simulink model "simulation_scalar_robustness"  (R2021b)
settings: Solver=VariableStepAuto  StartTime=0.0  StopTime=20  MaxStep=0.01  RelTol=1e-3
values from neighbouring files (symbols this model uses):
  Delta = [1.9 0 -0.5 0 0.3 0 0.8 1.2 0 0 0 0 ... (25 elements, 5x5)]    [robustness.mat]    (also in test_URSR.m = round(Delta,1))
  k43 = 0    [exception.mat]    (also in robustness.mat = 663.324958071; scalar.mat = 61.6408497202; scalar_net.m = sqrt(2)*omega43*sqrt(abs(M(4,3)/M(3,4))); scalar_net_CreationNewConnection.m = sqrt(2)*omega43*sqrt(abs(M(4,3)/M(3,4))))
  k51 = 946.044396421    [exception.mat]    (also in robustness.mat = 146.385010942; scalar.mat = 259.670461528; scalar_net.m = sqrt(2)*omega51*sqrt(abs(M(5,1)/M(1,5))); scalar_net_CreationNewConnection.m = sqrt(2)*omega51*sqrt(abs(M(5,1)/M(1,5))))
  M = [-1.5 0 -0.7 0 17.9 0 -4.1 -6.8 0 0 0 0 ... (25 elements, 5x5)]    [exception.mat]    (also in nonscalar.mat = [-3.8 1.9 -4.5 0 0 0 -4.6 1.6 0 0 0 0 ... (25 elements, 5x5); nonscalar_net.m = round(M,1); nonscalar_net_general.m = sym('M',sum(n)); robustness.mat = [-8.5 0 -1.6 0 1.5 0 -5.3 -4.7 0 0 0 0 ... (25 elements, 5x5)
  omega43 = 50    [exception.mat]    (also in robustness.mat; scalar.mat; scalar_net.m = 200; scalar_net_CreationNewConnection.m)
  omega51 = 50    [exception.mat]    (also in robustness.mat = 70.7106781187; scalar.mat = 70.7106781187; scalar_net.m = sqrt(2) * omega_0; scalar_net_CreationNewConnection.m = sqrt(2) * omega_0)
  T = 2    [robustness.mat]    (also in test_URSR.m = -1/max(real(eig_M))*2*pi)
  x_0 = [1 1 1 1 1]    [exception.mat]    (also in nonscalar_net.m = ones(sum(n),1); robustness.mat; scalar.mat; scalar_net.m = ones(5,1))
settings Model: Creator=alber  LastModifiedBy=anobili

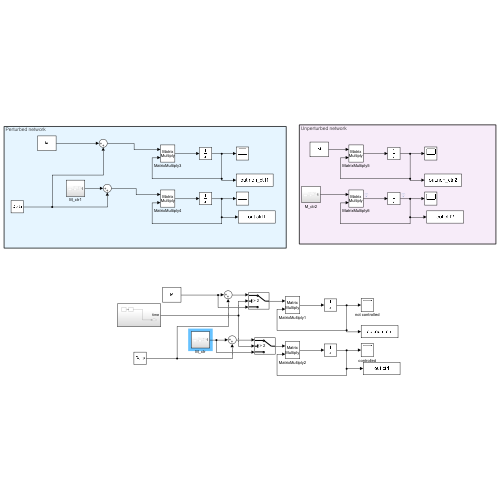
[thumbnail: Simulink's stored preview of the top-level diagram]
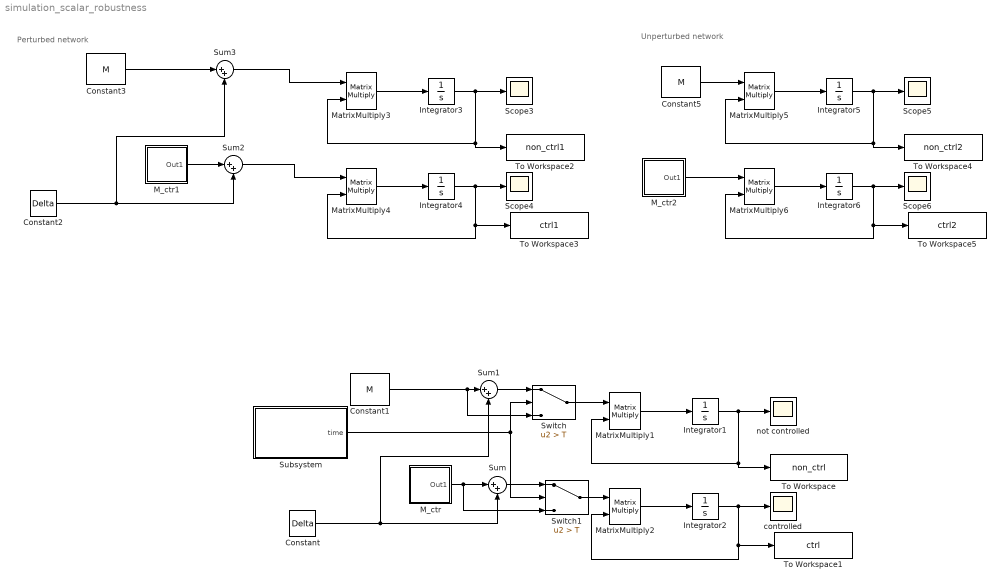
== system simulation_scalar_robustness ==
  note: Perturbed network
  note: Unperturbed network
  Constant : Constant  Value=Delta
  Constant1 : Constant  Value=M
  Constant2 : Constant  Value=Delta
  Constant3 : Constant  Value=M
  Constant5 : Constant  Value=M
  Integrator{1..6} (6 alike) : Integrator  InitialCondition=x_0
  M_ctr : Subsystem
  M_ctr1 : Subsystem
  M_ctr2 : Subsystem
  MatrixMultiply{1..6} (6 alike) : Product  Multiplication=Matrix(*)
  Scope{3..6} (4 alike) : Scope
  Subsystem : Subsystem
  Sum{,1..3} (4 alike) : Sum  Inputs=|++
  Switch : Switch  Criteria=u2 > Threshold  Threshold=T
  Switch1 : Switch  Criteria=u2 > Threshold  Threshold=T
  To Workspace : ToWorkspace  VariableName=non_ctrl  SaveFormat=Timeseries  SampleTime=-1
  To Workspace1 : ToWorkspace  VariableName=ctrl  SaveFormat=Timeseries  SampleTime=-1
  To Workspace2 : ToWorkspace  VariableName=non_ctrl1  SaveFormat=Timeseries  SampleTime=-1
  To Workspace3 : ToWorkspace  VariableName=ctrl1  SaveFormat=Timeseries  SampleTime=-1
  To Workspace4 : ToWorkspace  VariableName=non_ctrl2  SaveFormat=Timeseries  SampleTime=-1
  To Workspace5 : ToWorkspace  VariableName=ctrl2  SaveFormat=Timeseries  SampleTime=-1
  controlled : Scope
  not controlled : Scope
  wires:
  MatrixMultiply1/1 -> Integrator1/1
  Constant1/1 -> Switch/3, Sum1/1
  Integrator1/1 -> not controlled/1, To Workspace/1, MatrixMultiply1/2
  Integrator2/1 -> controlled/1, To Workspace1/1, MatrixMultiply2/2
  MatrixMultiply2/1 -> Integrator2/1
  Switch/1 -> MatrixMultiply1/1
  Switch1/1 -> MatrixMultiply2/1
  M_ctr/1(Out1) -> Switch1/3, Sum/1
  Subsystem/1(time) -> Switch1/2, Switch/2
  Constant/1 -> Sum1/2, Sum/2
  Sum1/1 -> Switch/1
  Sum/1 -> Switch1/1
  Sum2/1 -> MatrixMultiply4/1
  MatrixMultiply4/1 -> Integrator4/1
  Constant3/1 -> Sum3/1
  MatrixMultiply3/1 -> Integrator3/1
  Integrator3/1 -> Scope3/1, To Workspace2/1, MatrixMultiply3/2
  M_ctr1/1(Out1) -> Sum2/1
  Sum3/1 -> MatrixMultiply3/1
  Integrator4/1 -> Scope4/1, To Workspace3/1, MatrixMultiply4/2
  Constant2/1 -> Sum3/2, Sum2/2
  M_ctr2/1(Out1) -> MatrixMultiply6/1
  Integrator6/1 -> Scope6/1, To Workspace5/1, MatrixMultiply6/2
  Constant5/1 -> MatrixMultiply5/1
  Integrator5/1 -> Scope5/1, To Workspace4/1, MatrixMultiply5/2
  MatrixMultiply5/1 -> Integrator5/1
  MatrixMultiply6/1 -> Integrator6/1

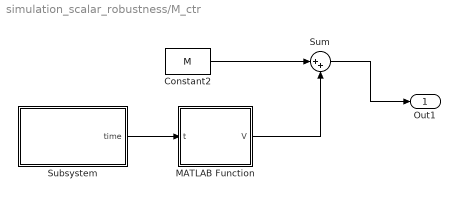
== system simulation_scalar_robustness/M_ctr ==
  Constant2 : Constant  Value=M
  MATLAB Function : MATLAB Function  TreatAsAtomicUnit=on
  Subsystem : Subsystem
  Sum : Sum  Inputs=|++
  Out1 : Outport
  wires:
  Constant2/1 -> Sum/1
  MATLAB Function/1(V) -> Sum/2
  Subsystem/1(time) -> MATLAB Function/1(t)
  Sum/1 -> Out1/1

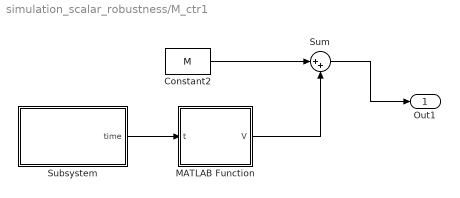
== system simulation_scalar_robustness/M_ctr1 ==
  Constant2 : Constant  Value=M
  MATLAB Function : MATLAB Function  TreatAsAtomicUnit=on
  Subsystem : Subsystem
  Sum : Sum  Inputs=|++
  Out1 : Outport
  wires:
  Constant2/1 -> Sum/1
  MATLAB Function/1(V) -> Sum/2
  Subsystem/1(time) -> MATLAB Function/1(t)
  Sum/1 -> Out1/1

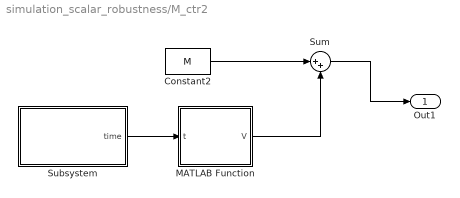
== system simulation_scalar_robustness/M_ctr2 ==
  Constant2 : Constant  Value=M
  MATLAB Function : MATLAB Function  TreatAsAtomicUnit=on
  Subsystem : Subsystem
  Sum : Sum  Inputs=|++
  Out1 : Outport
  wires:
  Constant2/1 -> Sum/1
  MATLAB Function/1(V) -> Sum/2
  Subsystem/1(time) -> MATLAB Function/1(t)
  Sum/1 -> Out1/1

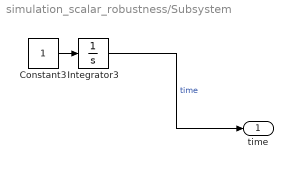
== system simulation_scalar_robustness/Subsystem ==
  Constant3 : Constant
  Integrator3 : Integrator
  time : Outport
  wires:
  Constant3/1 -> Integrator3/1
  Integrator3/1 -> time/1  "time"

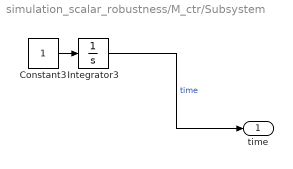
== system simulation_scalar_robustness/M_ctr/Subsystem ==
  Constant3 : Constant
  Integrator3 : Integrator
  time : Outport
  wires:
  Constant3/1 -> Integrator3/1
  Integrator3/1 -> time/1  "time"

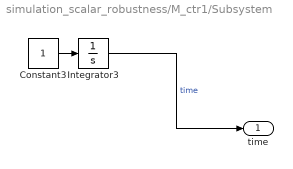
== system simulation_scalar_robustness/M_ctr1/Subsystem ==
  Constant3 : Constant
  Integrator3 : Integrator
  time : Outport
  wires:
  Constant3/1 -> Integrator3/1
  Integrator3/1 -> time/1  "time"

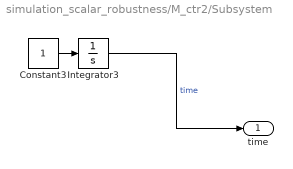
== system simulation_scalar_robustness/M_ctr2/Subsystem ==
  Constant3 : Constant
  Integrator3 : Integrator
  time : Outport
  wires:
  Constant3/1 -> Integrator3/1
  Integrator3/1 -> time/1  "time"

== matlab function simulation_scalar_robustness/M_ctr1/MATLAB Function ==
  data: t input; V output; omega43 parameter; k43 parameter; omega51 parameter; k51 parameter
function V = vibration(t, omega43, k43, omega51, k51)

V = zeros(5);
V(5,1) = k51*sin(omega51*t);
V(4,3) = k43*sin(omega43*t);

== matlab function simulation_scalar_robustness/M_ctr/MATLAB Function ==
  data: t input; V output; omega43 parameter; k43 parameter; omega51 parameter; k51 parameter
function V = vibration(t, omega43, k43, omega51, k51)

V = zeros(5);
V(5,1) = k51*sin(omega51*t);
V(4,3) = k43*sin(omega43*t);

== matlab function simulation_scalar_robustness/M_ctr2/MATLAB Function ==
  data: t input; V output; omega43 parameter; k43 parameter; omega51 parameter; k51 parameter
function V = vibration(t, omega43, k43, omega51, k51)

V = zeros(5);
V(5,1) = k51*sin(omega51*t);
V(4,3) = k43*sin(omega43*t);
